simulink model "canrx_0x1BF"  (R2022b)
settings: configuration reference "SLDD_CFG" (kept outside this file)
values from neighbouring files (symbols this model uses):
  K_CAN_GMLAN_RX_DEFAULT_TRB_CTRL_ENB_STAT = 0.0    [canrx_0x1BF.sldd]
  K_CAN_GMLAN_RX_DEFAULT_TRB_DUTY = 0.0    [canrx_0x1BF.sldd]
  K_CAN_GMLAN_RX_DEFAULT_TRB_ERR_MSG = 0.0    [canrx_0x1BF.sldd]
  K_CAN_GMLAN_RX_DEFAULT_TRB_POWER_OFF_ENB_STAT = 0.0    [canrx_0x1BF.sldd]
  K_CAN_GMLAN_RX_DEFAULT_VNT_ACT_POS = 0.0    [canrx_0x1BF.sldd]
  K_CAN_GMLAN_RX_INVALID_SELECT = 0.0    [canrx_0x1BF.sldd]
libraries: simulink x11
settings Model: DataDictionary=canrx_0x1BF.sldd  Creator=Castiel  LastModifiedBy=Castiel
settings ConfigSetRef: SourceName=SLDD_CFG

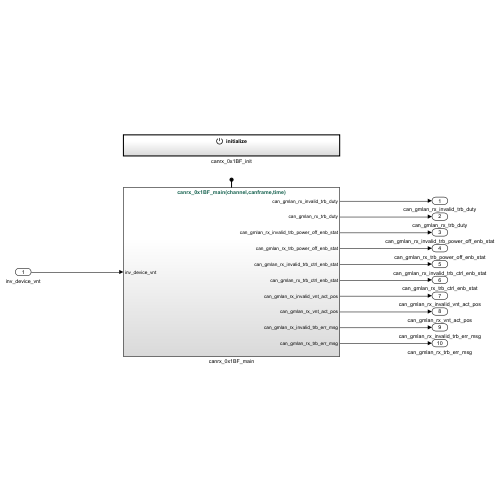
[thumbnail: Simulink's stored preview of the top-level diagram]
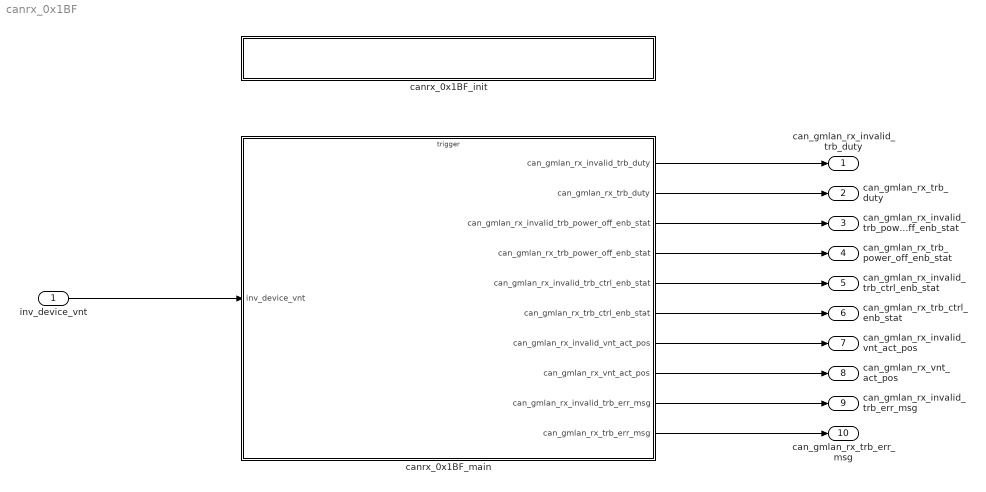
== system canrx_0x1BF ==
  inv_device_vnt : Inport
  canrx_0x1BF_init : Subsystem  TreatAsAtomicUnit=on
  canrx_0x1BF_main : Subsystem  TreatAsAtomicUnit=on
  can_gmlan_rx_invalid_trb_duty : Outport
  can_gmlan_rx_trb_duty : Outport  Port=2
  can_gmlan_rx_invalid_trb_power_off_enb_stat : Outport  Port=3
  can_gmlan_rx_trb_power_off_enb_stat : Outport  Port=4
  can_gmlan_rx_invalid_trb_ctrl_enb_stat : Outport  Port=5
  can_gmlan_rx_trb_ctrl_enb_stat : Outport  Port=6
  can_gmlan_rx_invalid_vnt_act_pos : Outport  Port=7
  can_gmlan_rx_vnt_act_pos : Outport  Port=8
  can_gmlan_rx_invalid_trb_err_msg : Outport  Port=9
  can_gmlan_rx_trb_err_msg : Outport  Port=10
  wires:
  inv_device_vnt/1 -> canrx_0x1BF_main/1(inv_device_vnt)
  canrx_0x1BF_main/1(can_gmlan_rx_invalid_trb_duty) -> can_gmlan_rx_invalid_trb_duty/1
  canrx_0x1BF_main/2(can_gmlan_rx_trb_duty) -> can_gmlan_rx_trb_duty/1
  canrx_0x1BF_main/3(can_gmlan_rx_invalid_trb_power_off_enb_stat) -> can_gmlan_rx_invalid_trb_power_off_enb_stat/1
  canrx_0x1BF_main/4(can_gmlan_rx_trb_power_off_enb_stat) -> can_gmlan_rx_trb_power_off_enb_stat/1
  canrx_0x1BF_main/5(can_gmlan_rx_invalid_trb_ctrl_enb_stat) -> can_gmlan_rx_invalid_trb_ctrl_enb_stat/1
  canrx_0x1BF_main/6(can_gmlan_rx_trb_ctrl_enb_stat) -> can_gmlan_rx_trb_ctrl_enb_stat/1
  canrx_0x1BF_main/7(can_gmlan_rx_invalid_vnt_act_pos) -> can_gmlan_rx_invalid_vnt_act_pos/1
  canrx_0x1BF_main/8(can_gmlan_rx_vnt_act_pos) -> can_gmlan_rx_vnt_act_pos/1
  canrx_0x1BF_main/9(can_gmlan_rx_invalid_trb_err_msg) -> can_gmlan_rx_invalid_trb_err_msg/1
  canrx_0x1BF_main/10(can_gmlan_rx_trb_err_msg) -> can_gmlan_rx_trb_err_msg/1

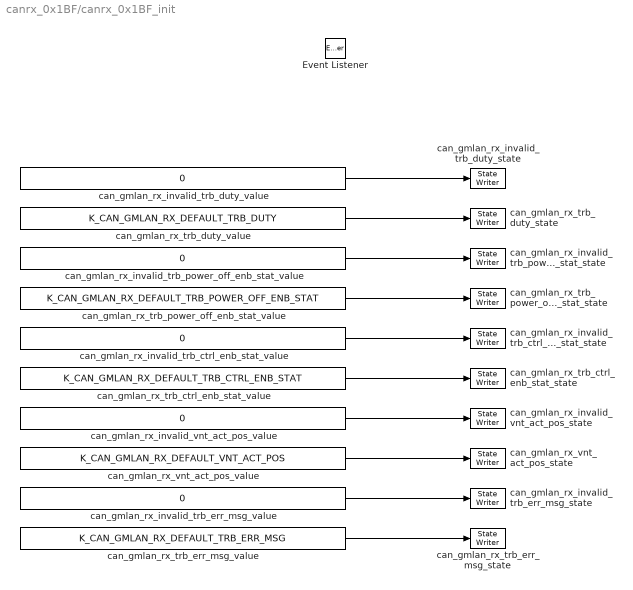
== system canrx_0x1BF/canrx_0x1BF_init ==
  Event Listener : EventListener  DisableCoverage=on  EventName=reset
  can_gmlan_rx_invalid_trb_ctrl_enb_stat_state : StateWriter  StateOwnerBlock=../../canrx_0x1BF_main/can_gmlan_rx_invalid_trb_ctrl_enb_stat
  can_gmlan_rx_invalid_trb_ctrl_enb_stat_value : Constant  Value=0  OutDataTypeStr=Inherit: Inherit via back propagation
  can_gmlan_rx_invalid_trb_duty_state : StateWriter  StateOwnerBlock=../../canrx_0x1BF_main/can_gmlan_rx_invalid_trb_duty
  can_gmlan_rx_invalid_trb_duty_value : Constant  Value=0  OutDataTypeStr=Inherit: Inherit via back propagation
  can_gmlan_rx_invalid_trb_err_msg_state : StateWriter  StateOwnerBlock=../../canrx_0x1BF_main/can_gmlan_rx_invalid_trb_err_msg
  can_gmlan_rx_invalid_trb_err_msg_value : Constant  Value=0  OutDataTypeStr=Inherit: Inherit via back propagation
  can_gmlan_rx_invalid_trb_power_off_enb_stat_state : StateWriter  StateOwnerBlock=../../canrx_0x1BF_main/can_gmlan_rx_invalid_trb_power_off_enb_stat
  can_gmlan_rx_invalid_trb_power_off_enb_stat_value : Constant  Value=0  OutDataTypeStr=Inherit: Inherit via back propagation
  can_gmlan_rx_invalid_vnt_act_pos_state : StateWriter  StateOwnerBlock=../../canrx_0x1BF_main/can_gmlan_rx_invalid_vnt_act_pos
  can_gmlan_rx_invalid_vnt_act_pos_value : Constant  Value=0  OutDataTypeStr=Inherit: Inherit via back propagation
  can_gmlan_rx_trb_ctrl_enb_stat_state : StateWriter  StateOwnerBlock=../../canrx_0x1BF_main/can_gmlan_rx_trb_ctrl_enb_stat
  can_gmlan_rx_trb_ctrl_enb_stat_value : Constant  Value=K_CAN_GMLAN_RX_DEFAULT_TRB_CTRL_ENB_STAT  OutDataTypeStr=Inherit: Inherit via back propagation
  can_gmlan_rx_trb_duty_state : StateWriter  StateOwnerBlock=../../canrx_0x1BF_main/can_gmlan_rx_trb_duty
  can_gmlan_rx_trb_duty_value : Constant  Value=K_CAN_GMLAN_RX_DEFAULT_TRB_DUTY  OutDataTypeStr=Inherit: Inherit via back propagation
  can_gmlan_rx_trb_err_msg_state : StateWriter  StateOwnerBlock=../../canrx_0x1BF_main/can_gmlan_rx_trb_err_msg
  can_gmlan_rx_trb_err_msg_value : Constant  Value=K_CAN_GMLAN_RX_DEFAULT_TRB_ERR_MSG  OutDataTypeStr=Inherit: Inherit via back propagation
  can_gmlan_rx_trb_power_off_enb_stat_state : StateWriter  StateOwnerBlock=../../canrx_0x1BF_main/can_gmlan_rx_trb_power_off_enb_stat
  can_gmlan_rx_trb_power_off_enb_stat_value : Constant  Value=K_CAN_GMLAN_RX_DEFAULT_TRB_POWER_OFF_ENB_STAT  OutDataTypeStr=Inherit: Inherit via back propagation
  can_gmlan_rx_vnt_act_pos_state : StateWriter  StateOwnerBlock=../../canrx_0x1BF_main/can_gmlan_rx_vnt_act_pos
  can_gmlan_rx_vnt_act_pos_value : Constant  Value=K_CAN_GMLAN_RX_DEFAULT_VNT_ACT_POS  OutDataTypeStr=Inherit: Inherit via back propagation
  wires:
  can_gmlan_rx_invalid_trb_duty_value/1 -> can_gmlan_rx_invalid_trb_duty_state/1
  can_gmlan_rx_trb_duty_value/1 -> can_gmlan_rx_trb_duty_state/1
  can_gmlan_rx_invalid_trb_power_off_enb_stat_value/1 -> can_gmlan_rx_invalid_trb_power_off_enb_stat_state/1
  can_gmlan_rx_trb_power_off_enb_stat_value/1 -> can_gmlan_rx_trb_power_off_enb_stat_state/1
  can_gmlan_rx_invalid_trb_ctrl_enb_stat_value/1 -> can_gmlan_rx_invalid_trb_ctrl_enb_stat_state/1
  can_gmlan_rx_trb_ctrl_enb_stat_value/1 -> can_gmlan_rx_trb_ctrl_enb_stat_state/1
  can_gmlan_rx_invalid_vnt_act_pos_value/1 -> can_gmlan_rx_invalid_vnt_act_pos_state/1
  can_gmlan_rx_vnt_act_pos_value/1 -> can_gmlan_rx_vnt_act_pos_state/1
  can_gmlan_rx_invalid_trb_err_msg_value/1 -> can_gmlan_rx_invalid_trb_err_msg_state/1
  can_gmlan_rx_trb_err_msg_value/1 -> can_gmlan_rx_trb_err_msg_state/1

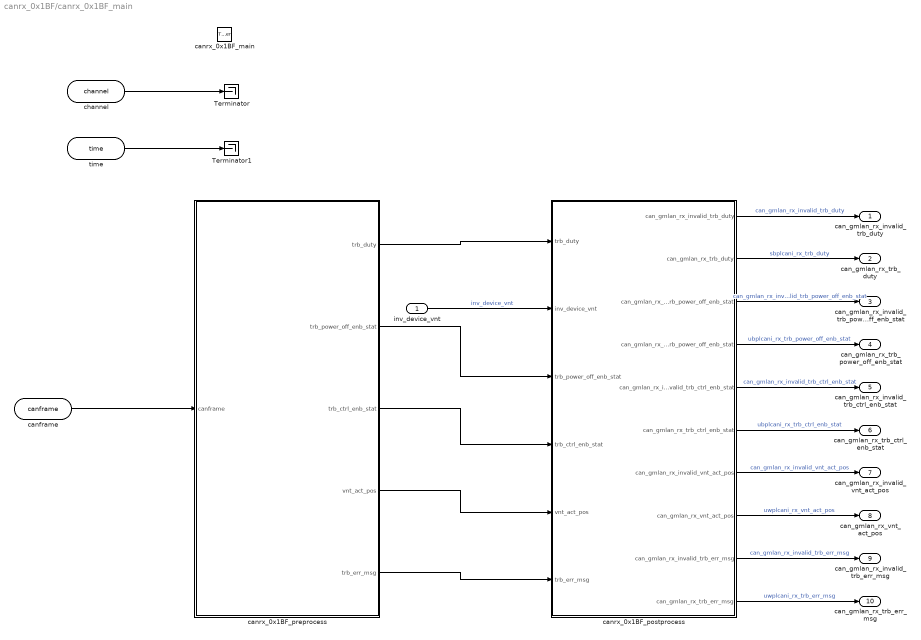
== system canrx_0x1BF/canrx_0x1BF_main ==
  inv_device_vnt : Inport
  canrx_0x1BF_main : TriggerPort  TriggerType=function-call  IsSimulinkFunction=on  FunctionName=canrx_0x1BF_main  FunctionVisibility=scoped  VariantControl=(inherit)
  Terminator : Terminator
  Terminator1 : Terminator
  canrx_0x1BF_postprocess : Subsystem  TreatAsAtomicUnit=on
      settings: RTWFcnNameOpts=Use subsystem name
  canrx_0x1BF_preprocess : Subsystem  TreatAsAtomicUnit=on
      settings: RTWFcnNameOpts=Use subsystem name
  channel : ArgIn  DisableCoverage=on  OutDataTypeStr=uint64  ArgumentName=channel
  canframe : ArgIn  DisableCoverage=on  Port=2  OutDataTypeStr=uint8  PortDimensions=8  ArgumentName=canframe
  time : ArgIn  DisableCoverage=on  Port=3  OutDataTypeStr=uint64  ArgumentName=time
  can_gmlan_rx_invalid_trb_duty : Outport
  can_gmlan_rx_trb_duty : Outport  Port=2
  can_gmlan_rx_invalid_trb_power_off_enb_stat : Outport  Port=3
  can_gmlan_rx_trb_power_off_enb_stat : Outport  Port=4
  can_gmlan_rx_invalid_trb_ctrl_enb_stat : Outport  Port=5
  can_gmlan_rx_trb_ctrl_enb_stat : Outport  Port=6
  can_gmlan_rx_invalid_vnt_act_pos : Outport  Port=7
  can_gmlan_rx_vnt_act_pos : Outport  Port=8
  can_gmlan_rx_invalid_trb_err_msg : Outport  Port=9
  can_gmlan_rx_trb_err_msg : Outport  Port=10
  wires:
  canframe/1 -> canrx_0x1BF_preprocess/1(canframe)
  channel/1 -> Terminator/1
  time/1 -> Terminator1/1
  canrx_0x1BF_preprocess/1(trb_duty) -> canrx_0x1BF_postprocess/1(trb_duty)
  canrx_0x1BF_preprocess/2(trb_power_off_enb_stat) -> canrx_0x1BF_postprocess/3(trb_power_off_enb_stat)
  canrx_0x1BF_preprocess/3(trb_ctrl_enb_stat) -> canrx_0x1BF_postprocess/4(trb_ctrl_enb_stat)
  canrx_0x1BF_preprocess/4(vnt_act_pos) -> canrx_0x1BF_postprocess/5(vnt_act_pos)
  canrx_0x1BF_preprocess/5(trb_err_msg) -> canrx_0x1BF_postprocess/6(trb_err_msg)
  inv_device_vnt/1 -> canrx_0x1BF_postprocess/2(inv_device_vnt)  "inv_device_vnt"
  canrx_0x1BF_postprocess/1(can_gmlan_rx_invalid_trb_duty) -> can_gmlan_rx_invalid_trb_duty/1  "can_gmlan_rx_invalid_trb_duty"
  canrx_0x1BF_postprocess/2(can_gmlan_rx_trb_duty) -> can_gmlan_rx_trb_duty/1  "sbplcani_rx_trb_duty"
  canrx_0x1BF_postprocess/3(can_gmlan_rx_invalid_trb_power_off_enb_stat) -> can_gmlan_rx_invalid_trb_power_off_enb_stat/1  "can_gmlan_rx_invalid_trb_power_off_enb_stat"
  canrx_0x1BF_postprocess/4(can_gmlan_rx_trb_power_off_enb_stat) -> can_gmlan_rx_trb_power_off_enb_stat/1  "ubplcani_rx_trb_power_off_enb_stat"
  canrx_0x1BF_postprocess/5(can_gmlan_rx_invalid_trb_ctrl_enb_stat) -> can_gmlan_rx_invalid_trb_ctrl_enb_stat/1  "can_gmlan_rx_invalid_trb_ctrl_enb_stat"
  canrx_0x1BF_postprocess/6(can_gmlan_rx_trb_ctrl_enb_stat) -> can_gmlan_rx_trb_ctrl_enb_stat/1  "ubplcani_rx_trb_ctrl_enb_stat"
  canrx_0x1BF_postprocess/7(can_gmlan_rx_invalid_vnt_act_pos) -> can_gmlan_rx_invalid_vnt_act_pos/1  "can_gmlan_rx_invalid_vnt_act_pos"
  canrx_0x1BF_postprocess/8(can_gmlan_rx_vnt_act_pos) -> can_gmlan_rx_vnt_act_pos/1  "uwplcani_rx_vnt_act_pos"
  canrx_0x1BF_postprocess/9(can_gmlan_rx_invalid_trb_err_msg) -> can_gmlan_rx_invalid_trb_err_msg/1  "can_gmlan_rx_invalid_trb_err_msg"
  canrx_0x1BF_postprocess/10(can_gmlan_rx_trb_err_msg) -> can_gmlan_rx_trb_err_msg/1  "uwplcani_rx_trb_err_msg"

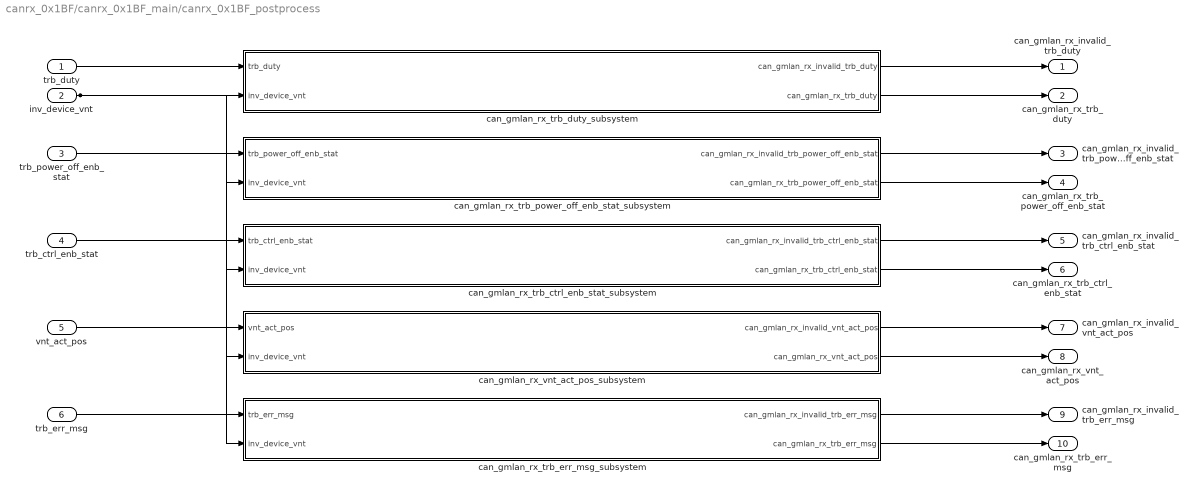
== system canrx_0x1BF/canrx_0x1BF_main/canrx_0x1BF_postprocess ==
  trb_duty : Inport
  inv_device_vnt : Inport  Port=2
  trb_power_off_enb_stat : Inport  Port=3
  trb_ctrl_enb_stat : Inport  Port=4
  vnt_act_pos : Inport  Port=5
  trb_err_msg : Inport  Port=6
  can_gmlan_rx_trb_ctrl_enb_stat_subsystem : Subsystem  TreatAsAtomicUnit=on
      settings: RTWFcnNameOpts=Use subsystem name
  can_gmlan_rx_trb_duty_subsystem : Subsystem  TreatAsAtomicUnit=on
      settings: RTWFcnNameOpts=Use subsystem name
  can_gmlan_rx_trb_err_msg_subsystem : Subsystem  TreatAsAtomicUnit=on
      settings: RTWFcnNameOpts=Use subsystem name
  can_gmlan_rx_trb_power_off_enb_stat_subsystem : Subsystem  TreatAsAtomicUnit=on
      settings: RTWFcnNameOpts=Use subsystem name
  can_gmlan_rx_vnt_act_pos_subsystem : Subsystem  TreatAsAtomicUnit=on
      settings: RTWFcnNameOpts=Use subsystem name
  can_gmlan_rx_invalid_trb_duty : Outport
  can_gmlan_rx_trb_duty : Outport  Port=2
  can_gmlan_rx_invalid_trb_power_off_enb_stat : Outport  Port=3
  can_gmlan_rx_trb_power_off_enb_stat : Outport  Port=4
  can_gmlan_rx_invalid_trb_ctrl_enb_stat : Outport  Port=5
  can_gmlan_rx_trb_ctrl_enb_stat : Outport  Port=6
  can_gmlan_rx_invalid_vnt_act_pos : Outport  Port=7
  can_gmlan_rx_vnt_act_pos : Outport  Port=8
  can_gmlan_rx_invalid_trb_err_msg : Outport  Port=9
  can_gmlan_rx_trb_err_msg : Outport  Port=10
  wires:
  trb_duty/1 -> can_gmlan_rx_trb_duty_subsystem/1(trb_duty)
  inv_device_vnt/1 -> can_gmlan_rx_trb_duty_subsystem/2(inv_device_vnt), can_gmlan_rx_trb_power_off_enb_stat_subsystem/2(inv_device_vnt), can_gmlan_rx_trb_ctrl_enb_stat_subsystem/2(inv_device_vnt), can_gmlan_rx_vnt_act_pos_subsystem/2(inv_device_vnt), can_gmlan_rx_trb_err_msg_subsystem/2(inv_device_vnt)
  can_gmlan_rx_trb_duty_subsystem/1(can_gmlan_rx_invalid_trb_duty) -> can_gmlan_rx_invalid_trb_duty/1
  can_gmlan_rx_trb_duty_subsystem/2(can_gmlan_rx_trb_duty) -> can_gmlan_rx_trb_duty/1
  trb_power_off_enb_stat/1 -> can_gmlan_rx_trb_power_off_enb_stat_subsystem/1(trb_power_off_enb_stat)
  can_gmlan_rx_trb_power_off_enb_stat_subsystem/1(can_gmlan_rx_invalid_trb_power_off_enb_stat) -> can_gmlan_rx_invalid_trb_power_off_enb_stat/1
  can_gmlan_rx_trb_power_off_enb_stat_subsystem/2(can_gmlan_rx_trb_power_off_enb_stat) -> can_gmlan_rx_trb_power_off_enb_stat/1
  trb_ctrl_enb_stat/1 -> can_gmlan_rx_trb_ctrl_enb_stat_subsystem/1(trb_ctrl_enb_stat)
  can_gmlan_rx_trb_ctrl_enb_stat_subsystem/1(can_gmlan_rx_invalid_trb_ctrl_enb_stat) -> can_gmlan_rx_invalid_trb_ctrl_enb_stat/1
  can_gmlan_rx_trb_ctrl_enb_stat_subsystem/2(can_gmlan_rx_trb_ctrl_enb_stat) -> can_gmlan_rx_trb_ctrl_enb_stat/1
  vnt_act_pos/1 -> can_gmlan_rx_vnt_act_pos_subsystem/1(vnt_act_pos)
  can_gmlan_rx_vnt_act_pos_subsystem/1(can_gmlan_rx_invalid_vnt_act_pos) -> can_gmlan_rx_invalid_vnt_act_pos/1
  can_gmlan_rx_vnt_act_pos_subsystem/2(can_gmlan_rx_vnt_act_pos) -> can_gmlan_rx_vnt_act_pos/1
  trb_err_msg/1 -> can_gmlan_rx_trb_err_msg_subsystem/1(trb_err_msg)
  can_gmlan_rx_trb_err_msg_subsystem/1(can_gmlan_rx_invalid_trb_err_msg) -> can_gmlan_rx_invalid_trb_err_msg/1
  can_gmlan_rx_trb_err_msg_subsystem/2(can_gmlan_rx_trb_err_msg) -> can_gmlan_rx_trb_err_msg/1

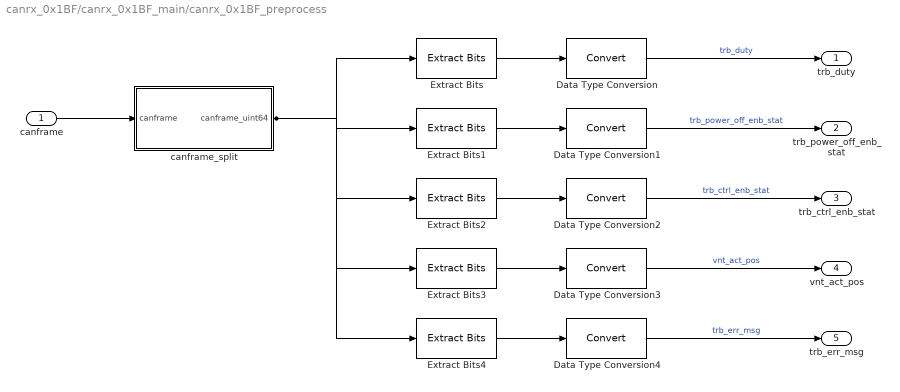
== system canrx_0x1BF/canrx_0x1BF_main/canrx_0x1BF_preprocess ==
  canframe : Inport
  Data Type Conversion{,1..4} (5 alike) : DataTypeConversion  ConvertRealWorld=Stored Integer (SI)  SaturateOnIntegerOverflow=off  RndMeth=Floor
  Extract Bits : simulink/Logic and Bit Operations/Extract Bits  bitsToExtract=Range of bits  numBits=8  bitIdxRange=[48 55]  outScalingMode=Treat bit field as an integer
  Extract Bits1 : simulink/Logic and Bit Operations/Extract Bits  bitsToExtract=Range of bits  numBits=8  bitIdxRange=[42 42]  outScalingMode=Treat bit field as an integer
  Extract Bits2 : simulink/Logic and Bit Operations/Extract Bits  bitsToExtract=Range of bits  numBits=8  bitIdxRange=[41 41]  outScalingMode=Treat bit field as an integer
  Extract Bits3 : simulink/Logic and Bit Operations/Extract Bits  bitsToExtract=Range of bits  numBits=8  bitIdxRange=[24 33]  outScalingMode=Treat bit field as an integer
  Extract Bits4 : simulink/Logic and Bit Operations/Extract Bits  bitsToExtract=Range of bits  numBits=8  bitIdxRange=[8 23]  outScalingMode=Treat bit field as an integer
  canframe_split : Subsystem
  trb_duty : Outport
  trb_power_off_enb_stat : Outport  Port=2
  trb_ctrl_enb_stat : Outport  Port=3
  vnt_act_pos : Outport  Port=4
  trb_err_msg : Outport  Port=5
  wires:
  canframe/1 -> canframe_split/1(canframe)
  canframe_split/1(canframe_uint64) -> Extract Bits/1, Extract Bits1/1, Extract Bits2/1, Extract Bits3/1, Extract Bits4/1
  Extract Bits/1 -> Data Type Conversion/1
  Data Type Conversion/1 -> trb_duty/1  "trb_duty"
  Extract Bits1/1 -> Data Type Conversion1/1
  Data Type Conversion1/1 -> trb_power_off_enb_stat/1  "trb_power_off_enb_stat"
  Extract Bits2/1 -> Data Type Conversion2/1
  Data Type Conversion2/1 -> trb_ctrl_enb_stat/1  "trb_ctrl_enb_stat"
  Extract Bits3/1 -> Data Type Conversion3/1
  Data Type Conversion3/1 -> vnt_act_pos/1  "vnt_act_pos"
  Extract Bits4/1 -> Data Type Conversion4/1
  Data Type Conversion4/1 -> trb_err_msg/1  "trb_err_msg"

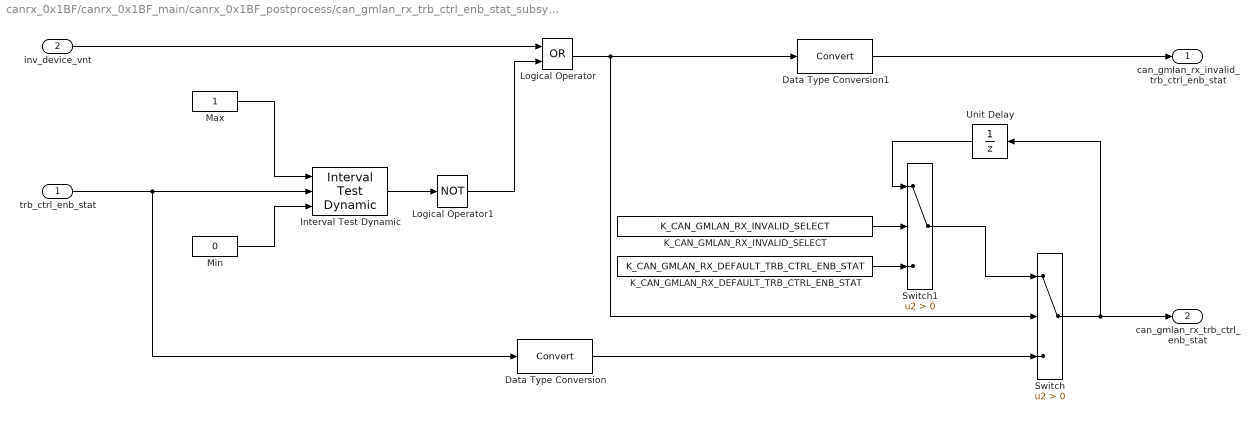
== system canrx_0x1BF/canrx_0x1BF_main/canrx_0x1BF_postprocess/can_gmlan_rx_trb_ctrl_enb_stat_subsystem ==
  trb_ctrl_enb_stat : Inport
  inv_device_vnt : Inport  Port=2
  Data Type Conversion : DataTypeConversion  ConvertRealWorld=Stored Integer (SI)  SaturateOnIntegerOverflow=off  RndMeth=Floor
  Data Type Conversion1 : DataTypeConversion  ConvertRealWorld=Stored Integer (SI)  SaturateOnIntegerOverflow=off  RndMeth=Floor
  Interval Test Dynamic : simulink/Logic and Bit Operations/Interval Test Dynamic  IntervalClosedRight=on  IntervalClosedLeft=on  OutDataTypeStr=boolean
  K_CAN_GMLAN_RX_DEFAULT_TRB_CTRL_ENB_STAT : Constant  Value=K_CAN_GMLAN_RX_DEFAULT_TRB_CTRL_ENB_STAT  OutDataTypeStr=Inherit: Inherit via back propagation
  K_CAN_GMLAN_RX_INVALID_SELECT : Constant  Value=K_CAN_GMLAN_RX_INVALID_SELECT  OutDataTypeStr=Inherit: Inherit via back propagation
  Logical Operator : Logic  Operator=OR  AllPortsSameDT=off  OutDataTypeStr=boolean
  Logical Operator1 : Logic  Operator=NOT  AllPortsSameDT=off  OutDataTypeStr=boolean
  Max : Constant  OutDataTypeStr=Inherit: Inherit via back propagation
  Min : Constant  Value=0  OutDataTypeStr=Inherit: Inherit via back propagation
  Switch : Switch  Criteria=u2 > Threshold  SaturateOnIntegerOverflow=off  InputSameDT=off
  Switch1 : Switch  Criteria=u2 > Threshold  SaturateOnIntegerOverflow=off  InputSameDT=off
  Unit Delay : UnitDelay  SampleTime=-1  HasFrameUpgradeWarning=on
  can_gmlan_rx_invalid_trb_ctrl_enb_stat : Outport
  can_gmlan_rx_trb_ctrl_enb_stat : Outport  Port=2
  wires:
  Data Type Conversion1/1 -> can_gmlan_rx_invalid_trb_ctrl_enb_stat/1
  Switch1/1 -> Switch/1
  K_CAN_GMLAN_RX_DEFAULT_TRB_CTRL_ENB_STAT/1 -> Switch1/3
  K_CAN_GMLAN_RX_INVALID_SELECT/1 -> Switch1/2
  Unit Delay/1 -> Switch1/1
  Logical Operator/1 -> Switch/2, Data Type Conversion1/1
  Switch/1 -> can_gmlan_rx_trb_ctrl_enb_stat/1, Unit Delay/1
  inv_device_vnt/1 -> Logical Operator/1
  Logical Operator1/1 -> Logical Operator/2
  Interval Test Dynamic/1 -> Logical Operator1/1
  Data Type Conversion/1 -> Switch/3
  Min/1 -> Interval Test Dynamic/3
  Max/1 -> Interval Test Dynamic/1
  trb_ctrl_enb_stat/1 -> Data Type Conversion/1, Interval Test Dynamic/2

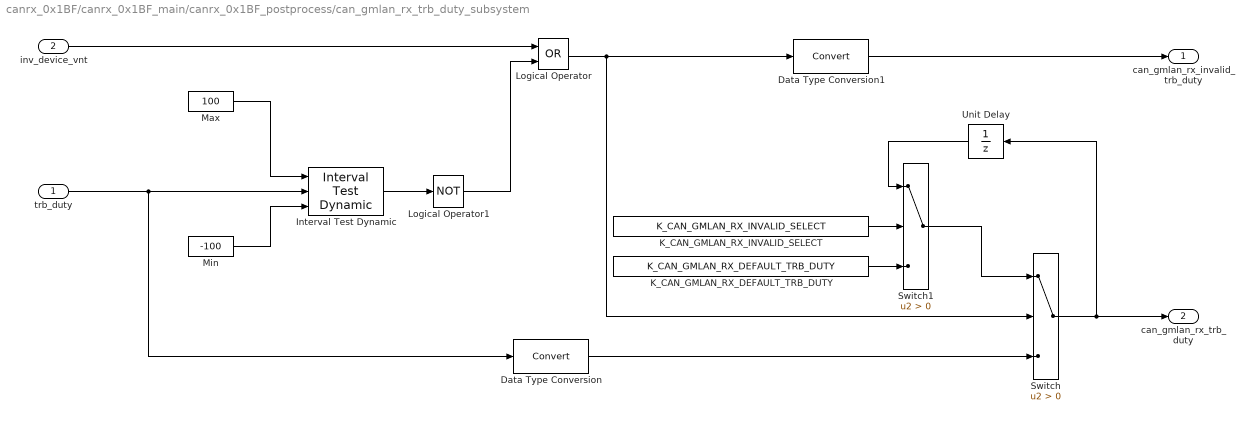
== system canrx_0x1BF/canrx_0x1BF_main/canrx_0x1BF_postprocess/can_gmlan_rx_trb_duty_subsystem ==
  trb_duty : Inport
  inv_device_vnt : Inport  Port=2
  Data Type Conversion : DataTypeConversion  ConvertRealWorld=Stored Integer (SI)  SaturateOnIntegerOverflow=off  RndMeth=Floor
  Data Type Conversion1 : DataTypeConversion  ConvertRealWorld=Stored Integer (SI)  SaturateOnIntegerOverflow=off  RndMeth=Floor
  Interval Test Dynamic : simulink/Logic and Bit Operations/Interval Test Dynamic  IntervalClosedRight=on  IntervalClosedLeft=on  OutDataTypeStr=boolean
  K_CAN_GMLAN_RX_DEFAULT_TRB_DUTY : Constant  Value=K_CAN_GMLAN_RX_DEFAULT_TRB_DUTY  OutDataTypeStr=Inherit: Inherit via back propagation
  K_CAN_GMLAN_RX_INVALID_SELECT : Constant  Value=K_CAN_GMLAN_RX_INVALID_SELECT  OutDataTypeStr=Inherit: Inherit via back propagation
  Logical Operator : Logic  Operator=OR  AllPortsSameDT=off  OutDataTypeStr=boolean
  Logical Operator1 : Logic  Operator=NOT  AllPortsSameDT=off  OutDataTypeStr=boolean
  Max : Constant  Value=100  OutDataTypeStr=Inherit: Inherit via back propagation
  Min : Constant  Value=-100  OutDataTypeStr=Inherit: Inherit via back propagation
  Switch : Switch  Criteria=u2 > Threshold  SaturateOnIntegerOverflow=off  InputSameDT=off
  Switch1 : Switch  Criteria=u2 > Threshold  SaturateOnIntegerOverflow=off  InputSameDT=off
  Unit Delay : UnitDelay  SampleTime=-1  HasFrameUpgradeWarning=on
  can_gmlan_rx_invalid_trb_duty : Outport
  can_gmlan_rx_trb_duty : Outport  Port=2
  wires:
  Data Type Conversion1/1 -> can_gmlan_rx_invalid_trb_duty/1
  Switch1/1 -> Switch/1
  K_CAN_GMLAN_RX_DEFAULT_TRB_DUTY/1 -> Switch1/3
  K_CAN_GMLAN_RX_INVALID_SELECT/1 -> Switch1/2
  Unit Delay/1 -> Switch1/1
  Logical Operator/1 -> Switch/2, Data Type Conversion1/1
  Switch/1 -> can_gmlan_rx_trb_duty/1, Unit Delay/1
  inv_device_vnt/1 -> Logical Operator/1
  Logical Operator1/1 -> Logical Operator/2
  Interval Test Dynamic/1 -> Logical Operator1/1
  Data Type Conversion/1 -> Switch/3
  Min/1 -> Interval Test Dynamic/3
  Max/1 -> Interval Test Dynamic/1
  trb_duty/1 -> Data Type Conversion/1, Interval Test Dynamic/2

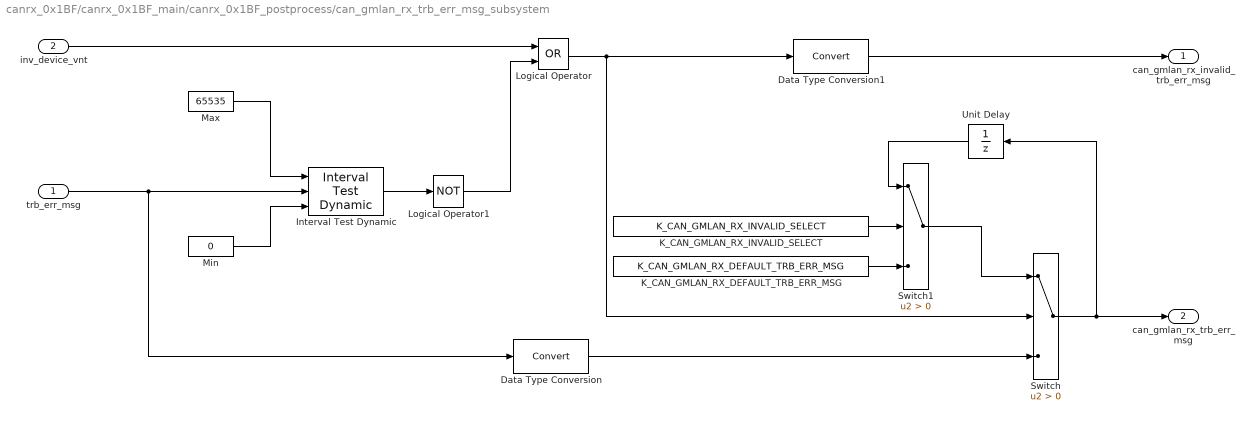
== system canrx_0x1BF/canrx_0x1BF_main/canrx_0x1BF_postprocess/can_gmlan_rx_trb_err_msg_subsystem ==
  trb_err_msg : Inport
  inv_device_vnt : Inport  Port=2
  Data Type Conversion : DataTypeConversion  ConvertRealWorld=Stored Integer (SI)  SaturateOnIntegerOverflow=off  RndMeth=Floor
  Data Type Conversion1 : DataTypeConversion  ConvertRealWorld=Stored Integer (SI)  SaturateOnIntegerOverflow=off  RndMeth=Floor
  Interval Test Dynamic : simulink/Logic and Bit Operations/Interval Test Dynamic  IntervalClosedRight=on  IntervalClosedLeft=on  OutDataTypeStr=boolean
  K_CAN_GMLAN_RX_DEFAULT_TRB_ERR_MSG : Constant  Value=K_CAN_GMLAN_RX_DEFAULT_TRB_ERR_MSG  OutDataTypeStr=Inherit: Inherit via back propagation
  K_CAN_GMLAN_RX_INVALID_SELECT : Constant  Value=K_CAN_GMLAN_RX_INVALID_SELECT  OutDataTypeStr=Inherit: Inherit via back propagation
  Logical Operator : Logic  Operator=OR  AllPortsSameDT=off  OutDataTypeStr=boolean
  Logical Operator1 : Logic  Operator=NOT  AllPortsSameDT=off  OutDataTypeStr=boolean
  Max : Constant  Value=65535  OutDataTypeStr=Inherit: Inherit via back propagation
  Min : Constant  Value=0  OutDataTypeStr=Inherit: Inherit via back propagation
  Switch : Switch  Criteria=u2 > Threshold  SaturateOnIntegerOverflow=off  InputSameDT=off
  Switch1 : Switch  Criteria=u2 > Threshold  SaturateOnIntegerOverflow=off  InputSameDT=off
  Unit Delay : UnitDelay  SampleTime=-1  HasFrameUpgradeWarning=on
  can_gmlan_rx_invalid_trb_err_msg : Outport
  can_gmlan_rx_trb_err_msg : Outport  Port=2
  wires:
  Data Type Conversion1/1 -> can_gmlan_rx_invalid_trb_err_msg/1
  Switch1/1 -> Switch/1
  K_CAN_GMLAN_RX_DEFAULT_TRB_ERR_MSG/1 -> Switch1/3
  K_CAN_GMLAN_RX_INVALID_SELECT/1 -> Switch1/2
  Unit Delay/1 -> Switch1/1
  Logical Operator/1 -> Switch/2, Data Type Conversion1/1
  Switch/1 -> can_gmlan_rx_trb_err_msg/1, Unit Delay/1
  inv_device_vnt/1 -> Logical Operator/1
  Logical Operator1/1 -> Logical Operator/2
  Interval Test Dynamic/1 -> Logical Operator1/1
  Data Type Conversion/1 -> Switch/3
  Min/1 -> Interval Test Dynamic/3
  Max/1 -> Interval Test Dynamic/1
  trb_err_msg/1 -> Data Type Conversion/1, Interval Test Dynamic/2

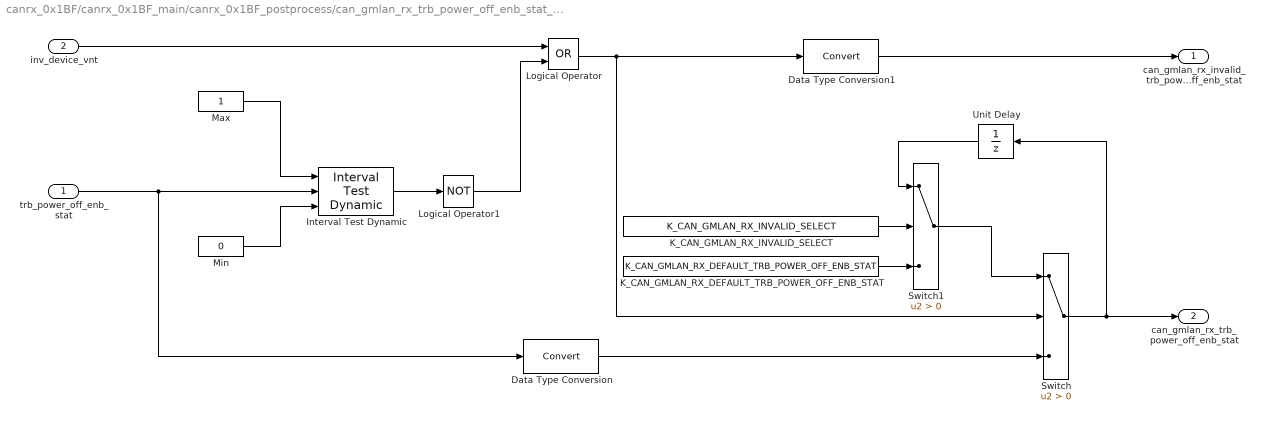
== system canrx_0x1BF/canrx_0x1BF_main/canrx_0x1BF_postprocess/can_gmlan_rx_trb_power_off_enb_stat_subsystem ==
  trb_power_off_enb_stat : Inport
  inv_device_vnt : Inport  Port=2
  Data Type Conversion : DataTypeConversion  ConvertRealWorld=Stored Integer (SI)  SaturateOnIntegerOverflow=off  RndMeth=Floor
  Data Type Conversion1 : DataTypeConversion  ConvertRealWorld=Stored Integer (SI)  SaturateOnIntegerOverflow=off  RndMeth=Floor
  Interval Test Dynamic : simulink/Logic and Bit Operations/Interval Test Dynamic  IntervalClosedRight=on  IntervalClosedLeft=on  OutDataTypeStr=boolean
  K_CAN_GMLAN_RX_DEFAULT_TRB_POWER_OFF_ENB_STAT : Constant  Value=K_CAN_GMLAN_RX_DEFAULT_TRB_POWER_OFF_ENB_STAT  OutDataTypeStr=Inherit: Inherit via back propagation
  K_CAN_GMLAN_RX_INVALID_SELECT : Constant  Value=K_CAN_GMLAN_RX_INVALID_SELECT  OutDataTypeStr=Inherit: Inherit via back propagation
  Logical Operator : Logic  Operator=OR  AllPortsSameDT=off  OutDataTypeStr=boolean
  Logical Operator1 : Logic  Operator=NOT  AllPortsSameDT=off  OutDataTypeStr=boolean
  Max : Constant  OutDataTypeStr=Inherit: Inherit via back propagation
  Min : Constant  Value=0  OutDataTypeStr=Inherit: Inherit via back propagation
  Switch : Switch  Criteria=u2 > Threshold  SaturateOnIntegerOverflow=off  InputSameDT=off
  Switch1 : Switch  Criteria=u2 > Threshold  SaturateOnIntegerOverflow=off  InputSameDT=off
  Unit Delay : UnitDelay  SampleTime=-1  HasFrameUpgradeWarning=on
  can_gmlan_rx_invalid_trb_power_off_enb_stat : Outport
  can_gmlan_rx_trb_power_off_enb_stat : Outport  Port=2
  wires:
  Data Type Conversion1/1 -> can_gmlan_rx_invalid_trb_power_off_enb_stat/1
  Switch1/1 -> Switch/1
  K_CAN_GMLAN_RX_DEFAULT_TRB_POWER_OFF_ENB_STAT/1 -> Switch1/3
  K_CAN_GMLAN_RX_INVALID_SELECT/1 -> Switch1/2
  Unit Delay/1 -> Switch1/1
  Logical Operator/1 -> Switch/2, Data Type Conversion1/1
  Switch/1 -> can_gmlan_rx_trb_power_off_enb_stat/1, Unit Delay/1
  inv_device_vnt/1 -> Logical Operator/1
  Logical Operator1/1 -> Logical Operator/2
  Interval Test Dynamic/1 -> Logical Operator1/1
  Data Type Conversion/1 -> Switch/3
  Min/1 -> Interval Test Dynamic/3
  Max/1 -> Interval Test Dynamic/1
  trb_power_off_enb_stat/1 -> Data Type Conversion/1, Interval Test Dynamic/2

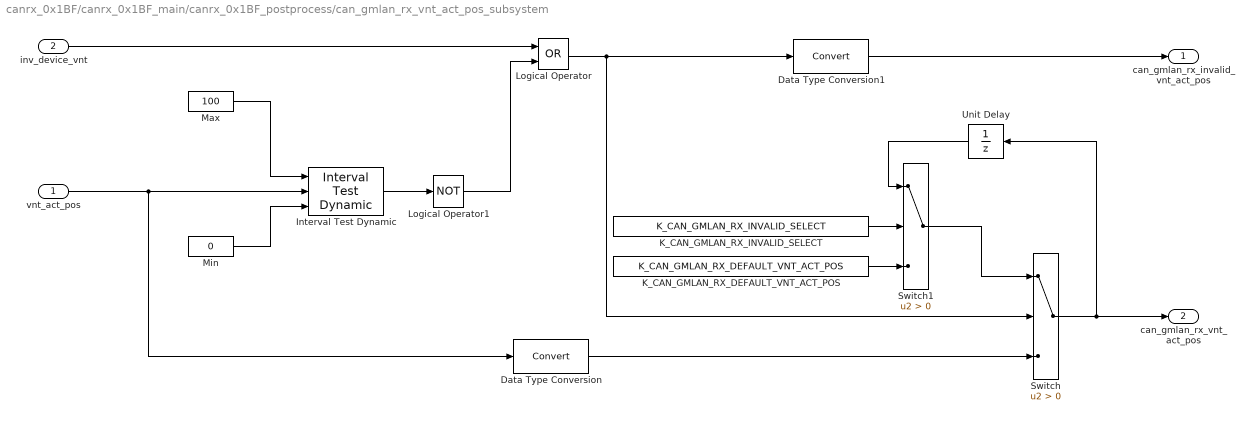
== system canrx_0x1BF/canrx_0x1BF_main/canrx_0x1BF_postprocess/can_gmlan_rx_vnt_act_pos_subsystem ==
  vnt_act_pos : Inport
  inv_device_vnt : Inport  Port=2
  Data Type Conversion : DataTypeConversion  ConvertRealWorld=Stored Integer (SI)  SaturateOnIntegerOverflow=off  RndMeth=Floor
  Data Type Conversion1 : DataTypeConversion  ConvertRealWorld=Stored Integer (SI)  SaturateOnIntegerOverflow=off  RndMeth=Floor
  Interval Test Dynamic : simulink/Logic and Bit Operations/Interval Test Dynamic  IntervalClosedRight=on  IntervalClosedLeft=on  OutDataTypeStr=boolean
  K_CAN_GMLAN_RX_DEFAULT_VNT_ACT_POS : Constant  Value=K_CAN_GMLAN_RX_DEFAULT_VNT_ACT_POS  OutDataTypeStr=Inherit: Inherit via back propagation
  K_CAN_GMLAN_RX_INVALID_SELECT : Constant  Value=K_CAN_GMLAN_RX_INVALID_SELECT  OutDataTypeStr=Inherit: Inherit via back propagation
  Logical Operator : Logic  Operator=OR  AllPortsSameDT=off  OutDataTypeStr=boolean
  Logical Operator1 : Logic  Operator=NOT  AllPortsSameDT=off  OutDataTypeStr=boolean
  Max : Constant  Value=100  OutDataTypeStr=Inherit: Inherit via back propagation
  Min : Constant  Value=0  OutDataTypeStr=Inherit: Inherit via back propagation
  Switch : Switch  Criteria=u2 > Threshold  SaturateOnIntegerOverflow=off  InputSameDT=off
  Switch1 : Switch  Criteria=u2 > Threshold  SaturateOnIntegerOverflow=off  InputSameDT=off
  Unit Delay : UnitDelay  SampleTime=-1  HasFrameUpgradeWarning=on
  can_gmlan_rx_invalid_vnt_act_pos : Outport
  can_gmlan_rx_vnt_act_pos : Outport  Port=2
  wires:
  Data Type Conversion1/1 -> can_gmlan_rx_invalid_vnt_act_pos/1
  Switch1/1 -> Switch/1
  K_CAN_GMLAN_RX_DEFAULT_VNT_ACT_POS/1 -> Switch1/3
  K_CAN_GMLAN_RX_INVALID_SELECT/1 -> Switch1/2
  Unit Delay/1 -> Switch1/1
  Logical Operator/1 -> Switch/2, Data Type Conversion1/1
  Switch/1 -> can_gmlan_rx_vnt_act_pos/1, Unit Delay/1
  inv_device_vnt/1 -> Logical Operator/1
  Logical Operator1/1 -> Logical Operator/2
  Interval Test Dynamic/1 -> Logical Operator1/1
  Data Type Conversion/1 -> Switch/3
  Min/1 -> Interval Test Dynamic/3
  Max/1 -> Interval Test Dynamic/1
  vnt_act_pos/1 -> Data Type Conversion/1, Interval Test Dynamic/2

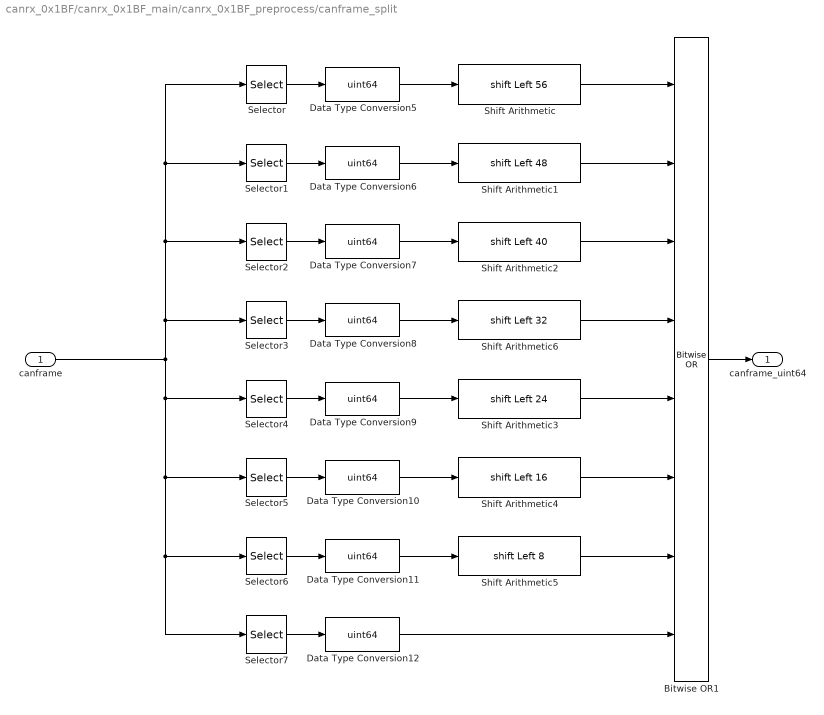
== system canrx_0x1BF/canrx_0x1BF_main/canrx_0x1BF_preprocess/canframe_split ==
  canframe : Inport
  Bitwise OR1 : simulink/Logic and Bit Operations/Bitwise Operator  logicop=OR  UseBitMask=off  NumInputPorts=8  BitMask=bin2dec('11011001')  BitMaskRealWorld=Stored Integer
  Data Type Conversion{5..12} (8 alike) : DataTypeConversion  OutDataTypeStr=uint64  ConvertRealWorld=Stored Integer (SI)  SaturateOnIntegerOverflow=off  RndMeth=Floor
  Selector : Selector  IndexMode=Zero-based  InputPortWidth=8  IndexOptions=Index vector (dialog)  Indices=0  OutputSizes=1
  Selector1 : Selector  IndexMode=Zero-based  InputPortWidth=8  IndexOptions=Index vector (dialog)  Indices=1  OutputSizes=1
  Selector2 : Selector  IndexMode=Zero-based  InputPortWidth=8  IndexOptions=Index vector (dialog)  Indices=2  OutputSizes=1
  Selector3 : Selector  IndexMode=Zero-based  InputPortWidth=8  IndexOptions=Index vector (dialog)  Indices=3  OutputSizes=1
  Selector4 : Selector  IndexMode=Zero-based  InputPortWidth=8  IndexOptions=Index vector (dialog)  Indices=4  OutputSizes=1
  Selector5 : Selector  IndexMode=Zero-based  InputPortWidth=8  IndexOptions=Index vector (dialog)  Indices=5  OutputSizes=1
  Selector6 : Selector  IndexMode=Zero-based  InputPortWidth=8  IndexOptions=Index vector (dialog)  Indices=6  OutputSizes=1
  Selector7 : Selector  IndexMode=Zero-based  InputPortWidth=8  IndexOptions=Index vector (dialog)  Indices=7  OutputSizes=1
  Shift Arithmetic : ArithShift  BitShiftNumber=56  BitShiftDirection=Left  DiagnosticForOORShift=Error
  Shift Arithmetic1 : ArithShift  BitShiftNumber=48  BitShiftDirection=Left  DiagnosticForOORShift=Error
  Shift Arithmetic2 : ArithShift  BitShiftNumber=40  BitShiftDirection=Left  DiagnosticForOORShift=Error
  Shift Arithmetic3 : ArithShift  BitShiftNumber=24  BitShiftDirection=Left  DiagnosticForOORShift=Error
  Shift Arithmetic4 : ArithShift  BitShiftNumber=16  BitShiftDirection=Left  DiagnosticForOORShift=Error
  Shift Arithmetic5 : ArithShift  BitShiftNumber=8  BitShiftDirection=Left  DiagnosticForOORShift=Error
  Shift Arithmetic6 : ArithShift  BitShiftNumber=32  BitShiftDirection=Left  DiagnosticForOORShift=Error
  canframe_uint64 : Outport
  wires:
  Bitwise OR1/1 -> canframe_uint64/1
  Data Type Conversion5/1 -> Shift Arithmetic/1
  Selector/1 -> Data Type Conversion5/1
  Selector1/1 -> Data Type Conversion6/1
  Data Type Conversion11/1 -> Shift Arithmetic5/1
  Shift Arithmetic5/1 -> Bitwise OR1/7
  Selector6/1 -> Data Type Conversion11/1
  Selector2/1 -> Data Type Conversion7/1
  Data Type Conversion10/1 -> Shift Arithmetic4/1
  Shift Arithmetic6/1 -> Bitwise OR1/4
  Data Type Conversion8/1 -> Shift Arithmetic6/1
  Shift Arithmetic1/1 -> Bitwise OR1/2
  Data Type Conversion7/1 -> Shift Arithmetic2/1
  Data Type Conversion12/1 -> Bitwise OR1/8
  Selector7/1 -> Data Type Conversion12/1
  Data Type Conversion9/1 -> Shift Arithmetic3/1
  Selector3/1 -> Data Type Conversion8/1
  Shift Arithmetic3/1 -> Bitwise OR1/5
  Selector5/1 -> Data Type Conversion10/1
  Shift Arithmetic4/1 -> Bitwise OR1/6
  Selector4/1 -> Data Type Conversion9/1
  Shift Arithmetic2/1 -> Bitwise OR1/3
  Shift Arithmetic/1 -> Bitwise OR1/1
  Data Type Conversion6/1 -> Shift Arithmetic1/1
  canframe/1 -> Selector/1, Selector1/1, Selector2/1, Selector3/1, Selector4/1, Selector7/1, Selector6/1, Selector5/1
